simulink model "testcamObj"  (R2018b)
settings: Solver=FixedStepAuto  StartTime=0.0  StopTime=0.5  FixedStep=0.025  RelTol=1e-3  EnableMultiTasking=on
settings Model: Creator=Andy  LastModifiedBy=barthal
settings SolverCC: PositivePriorityOrder=on
settings DataIOCC: SaveFormat=StructureWithTime
settings OptimizationCC: EnhancedBackFolding=on  PassReuseOutputArgsAs=Individual arguments  MaxStackSize=64  OptimizeBlockOrder=speed  DifferentSizesBufferReuse=on  OptimizationCustomize=off
settings DebuggingCC: ParameterTunabilityLossMsg=error
settings HardwareCC: ProdBitPerPointer=32  ProdBitPerSizeT=32  ProdBitPerPtrDiffT=32  ProdLargestAtomicInteger=Long  ProdLargestAtomicFloat=Double  ProdWordSize=32  ProdHWDeviceType=ARM Compatible->ARM Cortex
settings ModelReferenceCC: ModelReferenceNumInstancesAllowed=Single
settings SFSimCC: MATLABDynamicMemAlloc=off
settings RTWCC: SystemTargetFile=ert.tlc  HardwareBoard=Raspberry Pi  TLCOptions="-aInlineSetEventsForThisBaseRateFcn=TLC_FALSE -aSuppressMultiTaskScheduler=TLC_FALSE  -aRateBasedStepFcn=0"  GenCodeOnly=on  TemplateMakefile=ert_default_tmf  GenerateReport=on  Toolchain=GNU GCC Raspberry Pi  BuildConfiguration=Faster Runs  IncludeHyperlinkInReport=on  LaunchReport=on  GenerateTraceInfo=on  GenerateTraceReport=on  GenerateTraceReportSl=on  GenerateTraceReportSf=on  GenerateTraceReportEml=on
settings CodeAppCC: ForceParamTrailComments=on  IgnoreCustomStorageClasses=off  OperatorAnnotations=on  SimulinkDataObjDesc=on  SFDataObjDesc=on  InsertBlockDesc=on
settings ERTTargetCC: MatFileLogging=on  SupportVariableSizeSignals=on

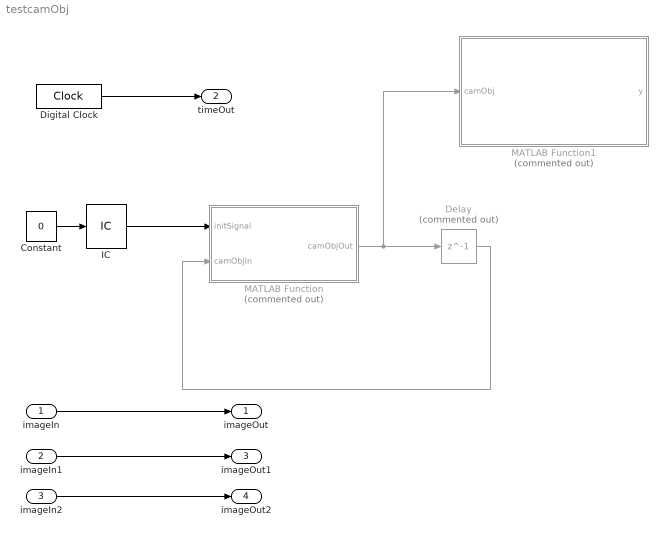
== system testcamObj ==
  imageIn : Inport  OutDataTypeStr=uint8  PortDimensions=[307200 3]
  imageIn1 : Inport  Port=2  OutDataTypeStr=uint8  PortDimensions=[307200]
  imageIn2 : Inport  Port=3  OutDataTypeStr=uint8  PortDimensions=[307200]
  Constant : Constant  Value=0
  Delay : Delay  Commented=on  DelayLength=1
  Digital Clock : DigitalClock  SampleTime=0.025
  IC : InitialCondition
  MATLAB Function : MATLAB Function  Commented=on  TreatAsAtomicUnit=on
  MATLAB Function1 : MATLAB Function  Commented=on  TreatAsAtomicUnit=on
  imageOut : Outport  OutDataTypeStr=uint8
  timeOut : Outport  Port=2
  imageOut1 : Outport  Port=3  OutDataTypeStr=uint8
  imageOut2 : Outport  Port=4  OutDataTypeStr=uint8
  wires:
  Constant/1 -> IC/1
  IC/1 -> MATLAB Function/1(initSignal)
  MATLAB Function/1(camObjOut) -> MATLAB Function1/1(camObj), Delay/1
  Delay/1 -> MATLAB Function/2(camObjIn)
  imageIn/1 -> imageOut/1
  Digital Clock/1 -> timeOut/1
  imageIn1/1 -> imageOut1/1
  imageIn2/1 -> imageOut2/1

== matlab function testcamObj/MATLAB Function1 ==
  data: camObj input; y output
function y = fcn(camObj)

y = step(camObj);

== matlab function testcamObj/MATLAB Function ==
  data: initSignal input; camObjOut output; camObjIn input
function camObjOut = openObj(initSignal,camObjIn)


if initSignal == 1
    camObjOut = imaq.VideoDevice;
else
    camObjOut = camObjIn;
end
